simulink library "DQN_Machines"  (R2023b)
settings: Solver=VariableStepAuto  StartTime=0.0  StopTime=10.0  RelTol=1e-3
undefined symbols (not defined in the file): DiscIntNeverNeededParam, N, SM, Ts
libraries: spsabctodq0Lib x2, spsdq0toabcLib x2
(part 3 of 5)

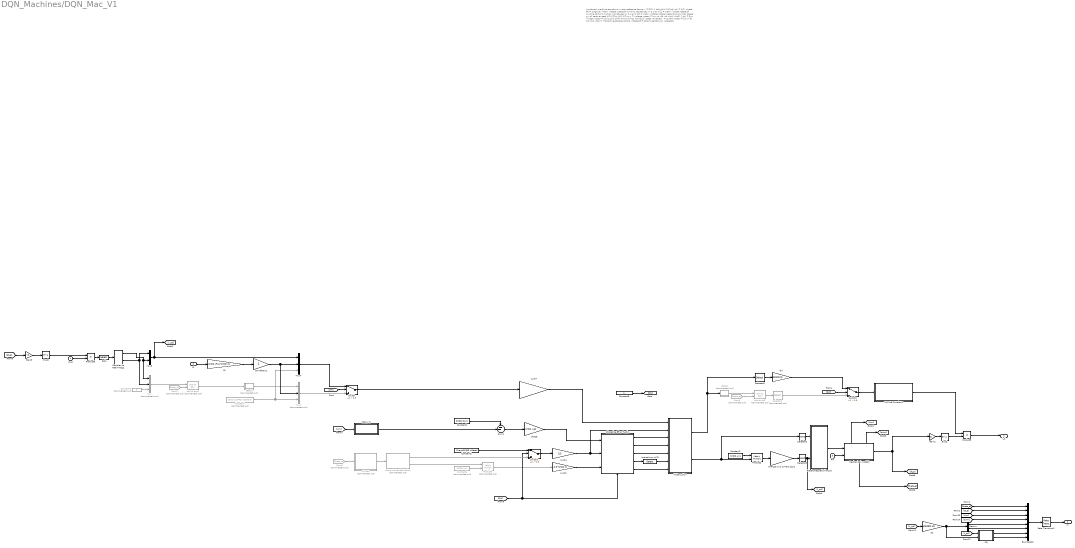
== system DQN_Machines/DQN_Mac_V1 ==
  note: Implement  machine equations in rotor reference frame:
      |   v = [R]*i + dphi/dt + [W]*phi
      | phi = [L]*i
      |
      | where:
      | [R] = diagonal matrix (nState,nState)of winding resistances in d q axis
      | [L] = matrix (nSate,nState)of winding self and mutual inductances in d q axis
      | [W] = matrix (nState,nState) depending on rotor speed wr,
      |       all zeros except W(1,2)=wr  W(2,1)=-wr
      |
      |   v = voltage vector      = [vq   vd   vfd   vkd   vkq1   (vkq2)  ]'
      | phi = flux linkage vector = [phiq phid phifd phikd phikq1 (phikq2)]' (state variables)
      |   i = current vector      = [iq   id   ifd   ikd   ikq1   (ikq2)  ]'
      |
      | if RotorType=Salient-Pole, nState=5
      | if RotorType=Round,        nState=6
  Vs_C : Inport
  Vf : Inport  Port=2
  Pm : Inport  Port=3
  1_Vb1 : Gain  Gain=-0.5*SMRD.Ib  SaturateOnIntegerOverflow=on  OutDataTypeStr=Inherit: Same as input  ParamDataTypeStr=Inherit: Same as input
  1_Vb4 : Gain  Gain=1/3  SaturateOnIntegerOverflow=on  OutDataTypeStr=Inherit: Same as input  ParamDataTypeStr=Inherit: Same as input
  1_Vb7 : Gain  Gain=SMRD.web/SMRD.Vb  SaturateOnIntegerOverflow=on  OutDataTypeStr=Inherit: Same as input  ParamDataTypeStr=Inherit: Same as input
  ABsel2 : Subsystem  Commented=on
  ABsel3 : Subsystem  Commented=on
  Bus Creator : BusCreator  Inputs=8
  Complex to Real-Imag1 : ComplexToRealImag
  Constant : Constant  Commented=on  Value=zeros(1,SMRD.nState-3)
  Constant1 : Constant  Value=SMRD.RLinv
  Constant2 : Constant  Value=3*eye(SMRD.nState)
  Constant4 : Constant  Commented=on  Value=SMRD.Linv
  Constant5 : Constant  Commented=on  Value=0
  Constant7 : Constant  Value=SMRD.Linv
  Constant8 : Constant
  Demux : Demux  Outputs=2
  Discretize BE or Tustin : Subsystem
      settings: PortSchema="{\"entries\":[{\"content\":{\"sides\":[{\"content\":{\"connectorIds\":[\"In1\",\"In2\",\"In3\"]},\"type\":\"ConnectorPlacement.EquallySpacedRectSide\",\"uuid\":\"a6b8bc68-dacc-495a-bf9e-1715fd4ce50f\"},{\"content\":{\"connectorIds\":[\"Out1\",\"Out2\",\"Out3\",\"Out4\",\"Out5\"],\"side\":\"RIGHT\"},\"type\":\"ConnectorPlacement.EquallySpacedRectSide\",\"uuid\":\"950ac892-f5e8-4081-8a8f-99bab3dfce2c\"},{\"content\":{\"side\":\"TOP\"},\"type\":\"ConnectorPlacement.EquallySpacedRectSide\",\"uuid\":\"9af2ed0d-ba89-43cd-9977-15872ca13b39\"},{\"content\":{\"connectorIds\":[\"In4\"],\"side\":\"BOTTOM\"},\"type\":\"ConnectorPlacement.EquallySpacedRectSide\",\"uuid\":\"e70e144b-23c4-40ad-9fe1-8550fd976efc\"}]},\"type\":\"ConnectorPlacement.EquallySpacedConnector\",\"uuid\":\"50b9889c-6d2c-45b1-ad8f-98a7760fa0a3\"}],\"packageUris\":[\"http://schema.mathworks.com/mf0/Connector/R2020b\"],\"version\":\"1.0\"}"
  Electromagnetic Torque : Subsystem
  Exp2 : Math
  Exp3 : Math
  From3 : From  Commented=on  GotoTag=theta_e
  From5 : From  Commented=on  GotoTag=theta_e
  From8 : From  Commented=on  GotoTag=theta_e
  Gain2 : Gain  Gain=1i
  Gain3 : Gain  Gain=-1i
  Ihistory_Flux : Subsystem
  MATLAB Function2 : MATLAB Function  TreatAsAtomicUnit=on  mask{N=SMRD.N}
      mask prompts: N "Harmonic order:"
  Matrix W : Subsystem
      settings: LibrarySourceBlock=spsSynchronousMachineModel/Discrete robust/Matrix W
  Mechanical model1 : Subsystem
      settings: LibrarySourceBlock=spsSynchronousMachineModel/Discrete Pm input trapezoidal  PortSchema="{\"entries\":[{\"content\":{\"sides\":[{\"content\":{\"connectorIds\":[\"In1\",\"In2\"]},\"type\":\"ConnectorPlacement.EquallySpacedRectSide\",\"uuid\":\"2381534f-5abc-4a8d-aa04-ab974f15f8a1\"},{\"content\":{\"connectorIds\":[\"Out1\"],\"side\":\"RIGHT\"},\"type\":\"ConnectorPlacement.EquallySpacedRectSide\",\"uuid\":\"4b91f832-d568-486f-91ee-7f5a07d19f05\"},{\"content\":{\"connectorIds\":[\"Out3\",\"Out4\"],\"side\":\"TOP\"},\"type\":\"ConnectorPlacement.EquallySpacedRectSide\",\"uuid\":\"94f23016-8fd9-49f0-81e0-4b44cc2bc22e\"},{\"content\":{\"connectorIds\":[\"Out2\"],\"side\":\"BOTTOM\"},\"type\":\"ConnectorPlacement.EquallySpacedRectSide\",\"uuid\":\"caf2a10e-4688-4978-a259-17b5afc46c0a\"}]},\"type\":\"ConnectorPlacement.EquallySpacedConnector\",\"uuid\":\"5998548e-4f7b-436e-b4ae-37de4e285cc4\"}],\"packageUris\":[\"http://schema.mathworks.com/mf0/Connector/R2020b\"],\"version\":\"1.0\"}"
  Mux : Mux  Commented=on  Inputs=3
  Mux1 : Mux  Commented=on  Inputs=[2 1 SMRD.nState-3]
  Mux3 : Mux  Inputs=2
  Mux4 : Mux  Inputs=[2 1 SMRD.nState-3]
  N1 : Gain  Gain=SMRD.Vfnp*SMRD.Vb  SaturateOnIntegerOverflow=on  OutDataTypeStr=Inherit: Same as input  ParamDataTypeStr=Inherit: Same as input
  N2 : Gain  Gain=1/SMRD.Vb  SaturateOnIntegerOverflow=on  OutDataTypeStr=Inherit: Same as input  ParamDataTypeStr=Inherit: Same as input
  PQ : Subsystem  AncestorBlock=spsSynchronousMachineModel/Discrete robust/Machine Measurements/PQ
  Product2 : Product  Multiplication=Matrix(*)  SaturateOnIntegerOverflow=on  OutDataTypeStr=Inherit: Same as first input
  Product4 : Product  Commented=on  Multiplication=Matrix(*)  SaturateOnIntegerOverflow=on  OutDataTypeStr=Inherit: Same as first input
  Product5 : Product
  Product6 : Product
  Rate Transition2 : RateTransition  Deterministic=off  OutPortSampleTime=Ts
  SM.VfGain1 : Gain
  Sel1 : Selector  NumberOfDimensions=2  InputPortWidth=3  IndexOptions=Index vector (dialog),Index vector (dialog)  Indices=1,2  OutputSizes=1
  Selector1 : Selector  Commented=on  InputPortWidth=3  IndexOptions=Index vector (dialog)  Indices=[1 2]  OutputSizes=1
  Selector2 : Selector  InputPortWidth=SMRD.nState  IndexOptions=Index vector (dialog)  Indices=[1 2]  OutputSizes=1
  Selector3 : Selector  InputPortWidth=SMRD.nState  IndexOptions=Index vector (dialog)  Indices=[1 2]  OutputSizes=1
  Selector5 : Selector  InputPortWidth=2  IndexOptions=Index vector (dialog)  Indices=[2 1]  OutputSizes=1
  Sum1 : Sum  Inputs=--|  SaturateOnIntegerOverflow=on
  Switch : Switch  Criteria=u2 > Threshold  Threshold=0.5  SaturateOnIntegerOverflow=off  InputSameDT=off
  Switch1 : Switch  Criteria=u2 > Threshold  Threshold=0.5  SaturateOnIntegerOverflow=off  InputSameDT=off
  Switch3 : Switch  Criteria=u2 > Threshold  Threshold=0.5  SaturateOnIntegerOverflow=off  InputSameDT=off
  abc to dq transformation : Subsystem  Commented=on
      settings: LibrarySourceBlock=|
      | spsSynchronousMachineModel/Discrete robust/abc to dq
      | transformation
  abc to dq0 : spsabctodq0Lib/abc to dq0  Commented=on  Alignment=90 degrees behind phase A axis
  change Iq Id current signs : Gain  Gain=SMRD.IqdSign
  dq0 to abc1 : spsdq0toabcLib/dq0 to abc  Commented=on  Alignment=90 degrees behind phase A axis
  ib4 : Gain  Gain=SMRD.Ib  SaturateOnIntegerOverflow=on  OutDataTypeStr=Inherit: Same as input  ParamDataTypeStr=Inherit: Same as input
  last column of D : Selector  NumberOfDimensions=2  InputPortWidth=3  IndexOptions=Index vector (dialog),Index vector (dialog)  Indices=[1:SMRD.nState],3  OutputSizes=1,1
  sin,cos : Subsystem  Commented=on
      settings: LibrarySourceBlock=spsSynchronousMachineModel/Discrete robust/sin,cos
  wbase : Gain  Gain=SMRD.web
  I_C : Outport  VectorParamsAs1DForOutWhenUnconnected=off
  m : Outport  Port=2  VectorParamsAs1DForOutWhenUnconnected=off
  wires:
  Vs_C/1 -> Product6/2  "vd,vq"
  sin,cos/1(sin,cos) -> abc to dq transformation/1(sin,cos)
  1_Vb1/1 -> Discretize BE or Tustin/3(C)
  last column of D/1 -> Ihistory_Flux/6(D(:,3))
  Discretize BE or Tustin/1(Ad) -> Ihistory_Flux/3(Ad)
  Discretize BE or Tustin/4(Dd) -> last column of D/1
  Electromagnetic Torque/1(Te) -> Mechanical model1/1(Te)
  Product2/1 -> change Iq Id current signs/1
  wbase/1 -> Discretize BE or Tustin/1(A)
  Discretize BE or Tustin/5(inv(I_Ts/2*A)) -> Ihistory_Flux/7(inv())
  Discretize BE or Tustin/2(Bd) -> Ihistory_Flux/4(Bd)
  Constant4/1 -> Product4/2  "Linv"
  Matrix W/1("[W]") -> Sum1/2
  Sum1/1 -> wbase/1  "A"
  Product4/1 -> 1_Vb1/1
  Ihistory_Flux/2(phi) -> Product2/2, Selector2/1
  Mechanical model1/2(theta_e) -> [theta_e]
  Mechanical model1/3(we) -> [wm]
  Pm/1 -> Mechanical model1/2(input)
  Constant7/1 -> Product2/1  "Linv"
  Constant2/1 -> Switch1/1
  ABsel3/1(Out1) -> Mux1/1
  Mux1/1 -> Switch/3  "u"
  Constant1/1 -> Sum1/1
  Vf/1 -> N1/1  "Vfd"
  Constant/1 -> Mux1/3, Mux4/3
  SM.VfGain1/1 -> Mux4/2, Mux1/2
  Mux4/1 -> Switch/1  "u"
  N1/1 -> SM.VfGain1/1  "Vfd"
  dq0 to abc1/1 -> ABsel3/1(v)
  abc to dq transformation/2(Ti (2x2)) -> Product4/1
  Switch1/1 -> 1_Vb4/1  "u"
  Ihistory_Flux/1(Ihyst) -> Selector5/1, ABsel2/1(v)  "I(k) = Linv*phi"
  MATLAB Function2/1(Vs_c) -> Product5/1
  Exp2/1 -> Product5/2
  Gain2/1 -> Exp2/1
  Switch/1 -> 1_Vb7/1
  Gain3/1 -> Exp3/1
  [dt_e] -> Gain3/1
  Product6/1 -> Sel1/1
  Exp3/1 -> Product6/1
  Sel1/1 -> Complex to Real-Imag1/1
  Mechanical model1/1(dtheta_e) -> [dt_e], Gain2/1
  Complex to Real-Imag1/2 -> Mux3/1, Mux/2
  Complex to Real-Imag1/1 -> Mux/1, Mux3/2
  Mux3/1 -> [v_qd], Mux4/1
  Switch3/1 -> MATLAB Function2/1(Vdq_vec)
  Mux/1 -> dq0 to abc1/1
  From3/1 -> dq0 to abc1/2
  Constant5/1 -> Mux/3
  1_Vb7/1 -> Ihistory_Flux/1(u)  "u"
  [SW] -> Switch/2
  Constant8/1 -> [SW]
  [SW] -> Switch1/2, Discretize BE or Tustin/4(SW)
  abc to dq transformation/1(Tv (nx3)) -> Switch1/3
  Selector1/1 -> Switch3/3  "Linv"
  [SW] -> Switch3/2
  Selector5/1 -> ib4/1
  abc to dq0/1 -> Selector1/1
  ABsel2/1(I) -> abc to dq0/1
  ib4/1 -> Switch3/1
  From5/1 -> abc to dq0/2
  Product5/1 -> I_C/1
  1_Vb4/1 -> Ihistory_Flux/2(B), Discretize BE or Tustin/2(B)
  [wm] -> Matrix W/1(wr)
  From8/1 -> sin,cos/1(theta)
  Discretize BE or Tustin/3(Cd) -> Ihistory_Flux/5(Cd)
  Bus Creator/1 -> Rate Transition2/1
  [theta_e] -> Bus Creator/1  "Rotor electrical angle  theta (rad)"
  [dt_e] -> Bus Creator/2  "Rotor angle deviation  d_theta (rad)"
  [wm] -> Bus Creator/3  "Rotor speed  wm  (pu)"
  Rate Transition2/1 -> m/1
  [v_qd] -> N2/1
  [i_qd] -> PQ/1(Iqd)
  PQ/1(Peo) -> Bus Creator/7  "Output active power   Peo (pu)"
  PQ/2(Qeo) -> Bus Creator/8  "Output reactive power  Qeo (pu)"
  Mechanical model1/4(dwe) -> [dwm]
  [dwm] -> Bus Creator/4  "Rotor speed deviation  dw (pu)"
  change Iq Id current signs/1 -> Selector3/1
  Selector3/1 -> [i_qd], Electromagnetic Torque/2(iqd)
  Selector2/1 -> Electromagnetic Torque/1(phiqd)
  N2/1 -> PQ/2(Vqd), Demux/1  "Vfd"
  Demux/1 -> Bus Creator/5  "Stator voltage  vq (pu)"
  Demux/2 -> Bus Creator/6  "Stator voltage  vd (pu)"

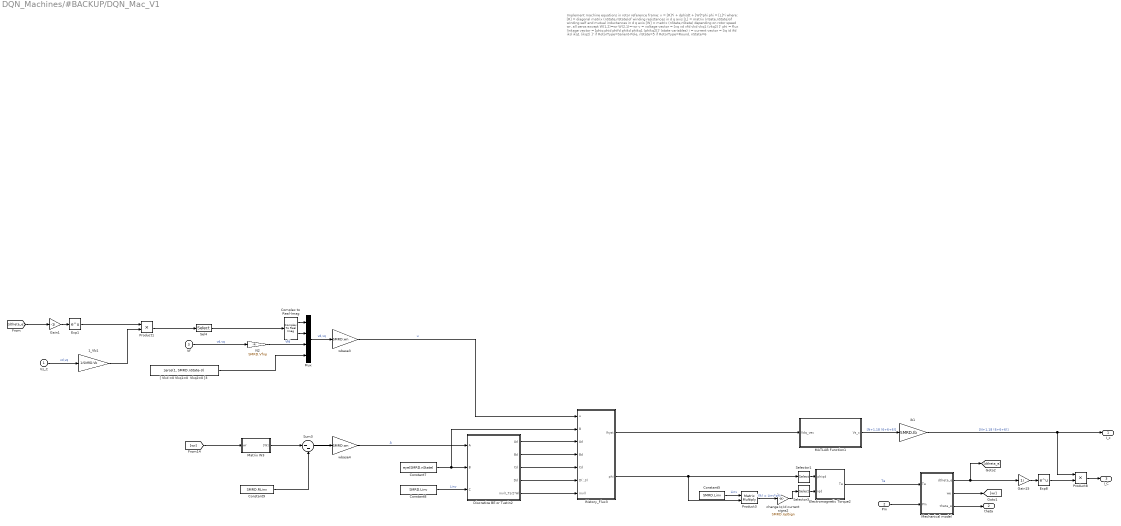
== system DQN_Machines/#BACKUP/DQN_Mac_V1 ==
  note: Implement  machine equations in rotor reference frame:
      |   v = [R]*i + dphi/dt + [W]*phi
      | phi = [L]*i
      |
      | where:
      | [R] = diagonal matrix (nState,nState)of winding resistances in d q axis
      | [L] = matrix (nSate,nState)of winding self and mutual inductances in d q axis
      | [W] = matrix (nState,nState) depending on rotor speed wr,
      |       all zeros except W(1,2)=wr  W(2,1)=-wr
      |
      |   v = voltage vector      = [vq   vd   vfd   vkd   vkq1   (vkq2)  ]'
      | phi = flux linkage vector = [phiq phid phifd phikd phikq1 (phikq2)]' (state variables)
      |   i = current vector      = [iq   id   ifd   ikd   ikq1   (ikq2)  ]'
      |
      | if RotorType=Salient-Pole, nState=5
      | if RotorType=Round,        nState=6
  Vs_C : Inport
  Pm : Inport  Port=2
  Vf : Inport  Port=3
  1_Vb1 : Gain  Gain=1/SMRD.Vb  SaturateOnIntegerOverflow=on  OutDataTypeStr=Inherit: Same as input  ParamDataTypeStr=Inherit: Same as input
  Complex to Real-Imag : ComplexToRealImag
  Constant5 : Constant  Value=SMRD.Linv
  Constant7 : Constant  Value=eye(SMRD.nState)
  Constant8 : Constant  Value=SMRD.Linv
  Constant9 : Constant  Value=SMRD.RLinv
  Discretize BE or Tustin2 : Subsystem  AncestorBlock="spsSynchronousMachineModel/Discrete robust/State Space Model/Discretize  BE or Tustin"
  Electromagnetic Torque2 : Subsystem
  Exp1 : Math
  Exp8 : Math
  Gain1 : Gain  Gain=-1i
  Gain15 : Gain  Gain=1i
  Ihistory_Flux3 : Subsystem  AncestorBlock=spsSynchronousMachineModel/Discrete robust/State Space Model/Ihistory_Flux
  MATLAB Function1 : MATLAB Function  TreatAsAtomicUnit=on  mask{N=SMRD.N}
      mask prompts: N "Harmonic order:"
  Matrix W3 : Subsystem
  Mechanical model : Subsystem
      settings: LibrarySourceBlock=spsSynchronousMachineModel/Discrete Pm input trapezoidal
  Mux : Mux
  N2 : Gain  Gain=SMRD.Vfnp  SaturateOnIntegerOverflow=on  OutDataTypeStr=Inherit: Same as input  ParamDataTypeStr=Inherit: Same as input
  Product1 : Product
  Product3 : Product  Multiplication=Matrix(*)  SaturateOnIntegerOverflow=on  OutDataTypeStr=Inherit: Same as first input
  Product8 : Product
  Sel4 : Selector  NumberOfDimensions=2  InputPortWidth=3  IndexOptions=Index vector (dialog),Index vector (dialog)  Indices=1,2  OutputSizes=1
  Selector1 : Selector  InputPortWidth=SMRD.nState  IndexOptions=Index vector (dialog)  Indices=[1 2]  OutputSizes=1
  Selector3 : Selector  InputPortWidth=SMRD.nState  IndexOptions=Index vector (dialog)  Indices=[1 2]  OutputSizes=1
  Sum3 : Sum  Inputs=|--  SaturateOnIntegerOverflow=on
  "[ Vkd =0 Vkq1=0  Vkq2=0 ]3" : Constant  Value=zeros(1, SMRD.nState-3)
  change Iq Id current signs2 : Gain  Gain=SMRD.IqdSign
  ib1 : Gain  Gain=SMRD.Ib  SaturateOnIntegerOverflow=on  OutDataTypeStr=Inherit: Same as input  ParamDataTypeStr=Inherit: Same as input
  wbase3 : Gain  Gain=SMRD.wn  SaturateOnIntegerOverflow=on  OutDataTypeStr=Inherit: Same as input  ParamDataTypeStr=Inherit: Same as input
  wbase4 : Gain  Gain=SMRD.wn  SaturateOnIntegerOverflow=on  OutDataTypeStr=Inherit: Same as input  ParamDataTypeStr=Inherit: Same as input
  I_c : Outport  VectorParamsAs1DForOutWhenUnconnected=off
  theta : Outport  Port=2  VectorParamsAs1DForOutWhenUnconnected=off
  I_C : Outport  Port=3  VectorParamsAs1DForOutWhenUnconnected=off
  wires:
  Selector3/1 -> Electromagnetic Torque2/2(iqd)
  Constant5/1 -> Product3/1  "Linv"
  Selector1/1 -> Electromagnetic Torque2/1(phiqd)
  Product3/1 -> change Iq Id current signs2/1  "I(k) = Linv*phi"
  Pm/1 -> Mechanical model/2(Pm)
  Electromagnetic Torque2/1(Te) -> Mechanical model/1(Te)  "Te"
  change Iq Id current signs2/1 -> Selector3/1
  MATLAB Function1/1(Vs_c) -> ib1/1  "[N+1,18 (6+6+6)]"
  ib1/1 -> Product8/1, I_c/1  "[N+1,18 (6+6+6)]"
  Sel4/1 -> Complex to Real-Imag/1
  Complex to Real-Imag/2 -> Mux/2
  Complex to Real-Imag/1 -> Mux/1
  N2/1 -> Mux/3  "Vfd"
  Mux/1 -> wbase3/1  "vd,vq"
  Mechanical model/3(theta_e) -> theta/1
  Mechanical model/2(we) -> [wr]
  Vs_C/1 -> 1_Vb1/1  "vd,vq"
  Vf/1 -> N2/1  "vd,vq"
  1_Vb1/1 -> Product1/2
  "[ Vkd =0 Vkq1=0  Vkq2=0 ]3"/1 -> Mux/4
  wbase3/1 -> Ihistory_Flux3/1(u)  "u"
  Discretize BE or Tustin2/4(Dd) -> Ihistory_Flux3/6(D(:,3))
  Discretize BE or Tustin2/5(inv(I_Ts/2*A)) -> Ihistory_Flux3/7(inv())
  Discretize BE or Tustin2/1(Ad) -> Ihistory_Flux3/3(Ad)
  Discretize BE or Tustin2/2(Bd) -> Ihistory_Flux3/4(Bd)
  Discretize BE or Tustin2/3(Cd) -> Ihistory_Flux3/5(Cd)
  Constant7/1 -> Ihistory_Flux3/2(B), Discretize BE or Tustin2/2(B)
  Sum3/1 -> wbase4/1
  Ihistory_Flux3/1(Ihyst) -> MATLAB Function1/1(Vdq_vec)
  Constant8/1 -> Discretize BE or Tustin2/3(C)  "Linv"
  [wr] -> Matrix W3/1(wr)
  Matrix W3/1("[W]") -> Sum3/1
  Constant9/1 -> Sum3/2
  wbase4/1 -> Discretize BE or Tustin2/1(A)  "A"
  Ihistory_Flux3/2(phi) -> Selector1/1, Product3/2
  Gain15/1 -> Exp8/1
  Product8/1 -> I_C/1
  Exp8/1 -> Product8/2
  Gain1/1 -> Exp1/1
  Exp1/1 -> Product1/1
  Product1/1 -> Sel4/1
  Mechanical model/1(dtheta_e) -> [dtheta_e], Gain15/1
  [dtheta_e] -> Gain1/1

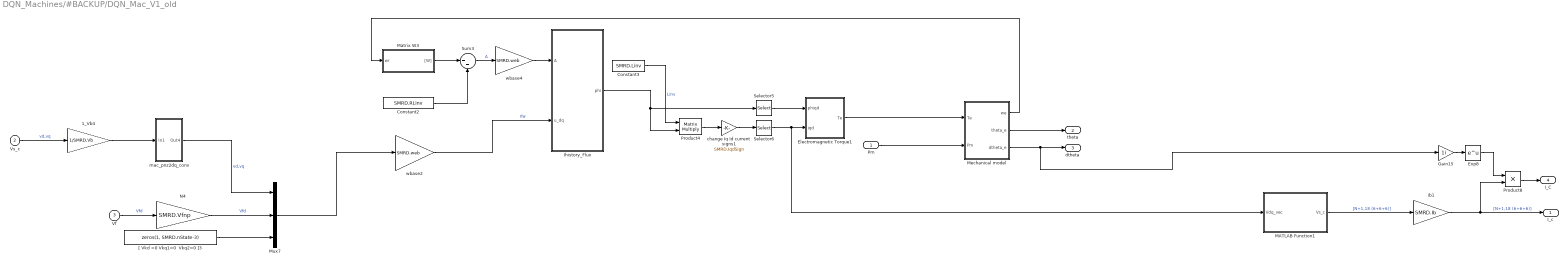
== system DQN_Machines/#BACKUP/DQN_Mac_V1_old ==
  Pm : Inport
  Vs_c : Inport  Port=2
  Vf : Inport  Port=3
  1_Vb4 : Gain  Gain=1/SMRD.Vb  SaturateOnIntegerOverflow=on  OutDataTypeStr=Inherit: Same as input  ParamDataTypeStr=Inherit: Same as input
  Constant2 : Constant  Value=SMRD.RLinv
  Constant3 : Constant  Value=SMRD.Linv
  Electromagnetic Torque1 : Subsystem
  Exp8 : Math
  Gain15 : Gain  Gain=1i
  Ihistory_Flux : Subsystem
  MATLAB Function1 : MATLAB Function  TreatAsAtomicUnit=on  mask{N=HRM}
      mask prompts: N "Harmonic order:"
  Matrix W3 : Subsystem  AncestorBlock=spsSynchronousMachineModel/Discrete robust/Matrix W
  Mechanical model : Subsystem  AncestorBlock=spsSynchronousMachineModel/Discrete Pm input trapezoidal
  Mux7 : Mux  Inputs="[ 2, 1,  (SMRD.nState-3) ]"
  N4 : Gain  Gain=SMRD.Vfnp  SaturateOnIntegerOverflow=on  OutDataTypeStr=Inherit: Same as input  ParamDataTypeStr=Inherit: Same as input
  Product4 : Product  Multiplication=Matrix(*)  SaturateOnIntegerOverflow=on  OutDataTypeStr=Inherit: Same as first input
  Product8 : Product
  Selector5 : Selector  InputPortWidth=SMRD.nState  IndexOptions=Index vector (dialog)  Indices=[1 2]  OutputSizes=1
  Selector6 : Selector  InputPortWidth=SMRD.nState  IndexOptions=Index vector (dialog)  Indices=[1 2]  OutputSizes=1
  Sum3 : Sum  Inputs=|--  SaturateOnIntegerOverflow=on
  "[ Vkd =0 Vkq1=0  Vkq2=0 ]3" : Constant  Value=zeros(1, SMRD.nState-3)
  change Iq Id current signs1 : Gain  Gain=SMRD.IqdSign
  ib1 : Gain  Gain=SMRD.Ib  SaturateOnIntegerOverflow=on  OutDataTypeStr=Inherit: Same as input  ParamDataTypeStr=Inherit: Same as input
  mac_pnz2dq_conv : Subsystem  mask{nrOut=1}
      mask prompts: nrOut "Number of outputs [{C}]"
      mask Display: disp(['{\color{red}\bf\fontsize{12}} [\{X_C\}]',newline,' MUX'], 'texmode','on');
  wbase2 : Gain  Gain=SMRD.web  SaturateOnIntegerOverflow=on  OutDataTypeStr=Inherit: Same as input  ParamDataTypeStr=Inherit: Same as input
  wbase4 : Gain  Gain=SMRD.web
  I_c : Outport  VectorParamsAs1DForOutWhenUnconnected=off
  theta : Outport  Port=2  VectorParamsAs1DForOutWhenUnconnected=off
  dtheta : Outport  Port=3  VectorParamsAs1DForOutWhenUnconnected=off
  I_C : Outport  Port=4  VectorParamsAs1DForOutWhenUnconnected=off
  wires:
  Sum3/1 -> wbase4/1  "A"
  Constant3/1 -> Product4/1  "Linv"
  Matrix W3/1("[W]") -> Sum3/1
  Mechanical model/2(theta_e) -> theta/1
  wbase4/1 -> Ihistory_Flux/1(A)
  Mechanical model/1(we) -> Matrix W3/1(wr)
  Ihistory_Flux/1(phi) -> Product4/2, Selector5/1
  MATLAB Function1/1(Vs_c) -> ib1/1  "[N+1,18 (6+6+6)]"
  Pm/1 -> Mechanical model/2(Pm)
  change Iq Id current signs1/1 -> Selector6/1
  Selector5/1 -> Electromagnetic Torque1/1(phiqd)
  Product4/1 -> change Iq Id current signs1/1
  Constant2/1 -> Sum3/2
  wbase2/1 -> Ihistory_Flux/2(u_dq)  "rlw"
  Electromagnetic Torque1/1(Te) -> Mechanical model/1(Te)
  "[ Vkd =0 Vkq1=0  Vkq2=0 ]3"/1 -> Mux7/3
  Vf/1 -> N4/1  "Vfd"
  Vs_c/1 -> 1_Vb4/1  "vd,vq"
  N4/1 -> Mux7/2  "Vfd"
  1_Vb4/1 -> mac_pnz2dq_conv/1(In1)
  Mux7/1 -> wbase2/1
  mac_pnz2dq_conv/1(Out4) -> Mux7/1  "vd,vq"
  Mechanical model/3(dtheta_e) -> Gain15/1, dtheta/1
  Selector6/1 -> MATLAB Function1/1(Vdq_vec), Electromagnetic Torque1/2(iqd)
  Product8/1 -> I_C/1
  Exp8/1 -> Product8/1
  ib1/1 -> Product8/2, I_c/1  "[N+1,18 (6+6+6)]"
  Gain15/1 -> Exp8/1

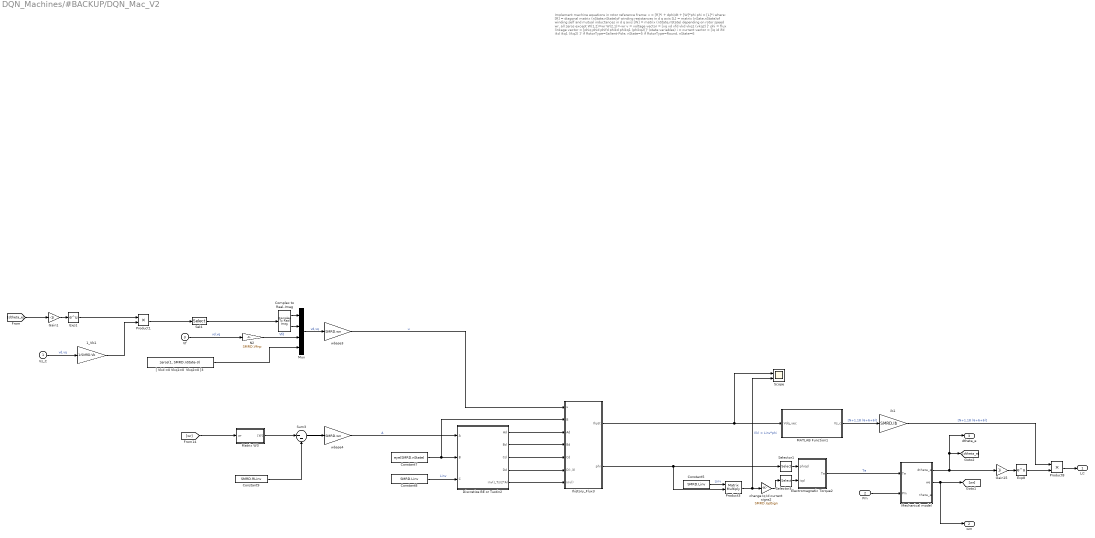
== system DQN_Machines/#BACKUP/DQN_Mac_V2 ==
  note: Implement  machine equations in rotor reference frame:
      |   v = [R]*i + dphi/dt + [W]*phi
      | phi = [L]*i
      |
      | where:
      | [R] = diagonal matrix (nState,nState)of winding resistances in d q axis
      | [L] = matrix (nSate,nState)of winding self and mutual inductances in d q axis
      | [W] = matrix (nState,nState) depending on rotor speed wr,
      |       all zeros except W(1,2)=wr  W(2,1)=-wr
      |
      |   v = voltage vector      = [vq   vd   vfd   vkd   vkq1   (vkq2)  ]'
      | phi = flux linkage vector = [phiq phid phifd phikd phikq1 (phikq2)]' (state variables)
      |   i = current vector      = [iq   id   ifd   ikd   ikq1   (ikq2)  ]'
      |
      | if RotorType=Salient-Pole, nState=5
      | if RotorType=Round,        nState=6
  Vs_C : Inport
  Pm : Inport  Port=2
  Vf : Inport  Port=3
  1_Vb1 : Gain  Gain=1/SMRD.Vb  SaturateOnIntegerOverflow=on  OutDataTypeStr=Inherit: Same as input  ParamDataTypeStr=Inherit: Same as input
  Complex to Real-Imag : ComplexToRealImag
  Constant5 : Constant  Value=SMRD.Linv
  Constant7 : Constant  Value=eye(SMRD.nState)
  Constant8 : Constant  Value=SMRD.Linv
  Constant9 : Constant  Value=SMRD.RLinv
  Discretize BE or Tustin2 : Subsystem  AncestorBlock="spsSynchronousMachineModel/Discrete robust/State Space Model/Discretize  BE or Tustin"
  Electromagnetic Torque2 : Subsystem
  Exp1 : Math
  Exp8 : Math
  Gain1 : Gain  Gain=-1i
  Gain15 : Gain  Gain=1i
  Ihistory_Flux3 : Subsystem  AncestorBlock=spsSynchronousMachineModel/Discrete robust/State Space Model/Ihistory_Flux
  MATLAB Function1 : MATLAB Function  TreatAsAtomicUnit=on  mask{N=SMRD.N}
      mask prompts: N "Harmonic order:"
  Matrix W3 : Subsystem
  Mechanical model : Subsystem
      settings: LibrarySourceBlock=spsSynchronousMachineModel/Discrete Pm input trapezoidal
  Mux : Mux
  N2 : Gain  Gain=SMRD.Vfnp  SaturateOnIntegerOverflow=on  OutDataTypeStr=Inherit: Same as input  ParamDataTypeStr=Inherit: Same as input
  Product1 : Product
  Product3 : Product  Multiplication=Matrix(*)  SaturateOnIntegerOverflow=on  OutDataTypeStr=Inherit: Same as first input
  Product8 : Product
  Scope : Scope  NumInputPorts=2
  Sel4 : Selector  NumberOfDimensions=2  InputPortWidth=3  IndexOptions=Index vector (dialog),Index vector (dialog)  Indices=1,2  OutputSizes=1
  Selector1 : Selector  InputPortWidth=SMRD.nState  IndexOptions=Index vector (dialog)  Indices=[1 2]  OutputSizes=1
  Selector3 : Selector  InputPortWidth=SMRD.nState  IndexOptions=Index vector (dialog)  Indices=[1 2]  OutputSizes=1
  Sum3 : Sum  Inputs=|--  SaturateOnIntegerOverflow=on
  "[ Vkd =0 Vkq1=0  Vkq2=0 ]3" : Constant  Value=zeros(1, SMRD.nState-3)
  change Iq Id current signs2 : Gain  Gain=SMRD.IqdSign
  ib1 : Gain  Gain=SMRD.Ib  SaturateOnIntegerOverflow=on  OutDataTypeStr=Inherit: Same as input  ParamDataTypeStr=Inherit: Same as input
  wbase3 : Gain  Gain=SMRD.wn  SaturateOnIntegerOverflow=on  OutDataTypeStr=Inherit: Same as input  ParamDataTypeStr=Inherit: Same as input
  wbase4 : Gain  Gain=SMRD.wn  SaturateOnIntegerOverflow=on  OutDataTypeStr=Inherit: Same as input  ParamDataTypeStr=Inherit: Same as input
  I_C : Outport  VectorParamsAs1DForOutWhenUnconnected=off
  wm : Outport  Port=2  VectorParamsAs1DForOutWhenUnconnected=off
  dtheta_e : Outport  Port=3  VectorParamsAs1DForOutWhenUnconnected=off
  wires:
  [dtheta_e] -> Gain1/1
  Mechanical model/1(dtheta_e) -> Gain15/1, dtheta_e/1, [dtheta_e]
  Product1/1 -> Sel4/1
  Exp1/1 -> Product1/1
  Gain1/1 -> Exp1/1
  Exp8/1 -> Product8/2
  Product8/1 -> I_C/1
  Gain15/1 -> Exp8/1
  Ihistory_Flux3/2(phi) -> Product3/2, Selector1/1
  wbase4/1 -> Discretize BE or Tustin2/1(A)  "A"
  Constant9/1 -> Sum3/2
  Matrix W3/1("[W]") -> Sum3/1
  [wr] -> Matrix W3/1(wr)
  Constant8/1 -> Discretize BE or Tustin2/3(C)  "Linv"
  Sum3/1 -> wbase4/1
  Constant7/1 -> Discretize BE or Tustin2/2(B), Ihistory_Flux3/2(B)
  Discretize BE or Tustin2/3(Cd) -> Ihistory_Flux3/5(Cd)
  Discretize BE or Tustin2/2(Bd) -> Ihistory_Flux3/4(Bd)
  Discretize BE or Tustin2/1(Ad) -> Ihistory_Flux3/3(Ad)
  Discretize BE or Tustin2/5(inv(I_Ts/2*A)) -> Ihistory_Flux3/7(inv())
  Discretize BE or Tustin2/4(Dd) -> Ihistory_Flux3/6(D(:,3))
  wbase3/1 -> Ihistory_Flux3/1(u)  "u"
  "[ Vkd =0 Vkq1=0  Vkq2=0 ]3"/1 -> Mux/4
  1_Vb1/1 -> Product1/2
  Vf/1 -> N2/1  "vd,vq"
  Vs_C/1 -> 1_Vb1/1  "vd,vq"
  Mechanical model/2(we) -> wm/1, [wr]
  Mux/1 -> wbase3/1  "vd,vq"
  N2/1 -> Mux/3  "Vfd"
  Complex to Real-Imag/1 -> Mux/1
  Complex to Real-Imag/2 -> Mux/2
  Sel4/1 -> Complex to Real-Imag/1
  ib1/1 -> Product8/1  "[N+1,18 (6+6+6)]"
  MATLAB Function1/1(Vs_c) -> ib1/1  "[N+1,18 (6+6+6)]"
  change Iq Id current signs2/1 -> Selector3/1
  Electromagnetic Torque2/1(Te) -> Mechanical model/1(Te)  "Te"
  Pm/1 -> Mechanical model/2(Pm)
  Product3/1 -> Scope/2, change Iq Id current signs2/1  "I(k) = Linv*phi"
  Selector1/1 -> Electromagnetic Torque2/1(phiqd)
  Constant5/1 -> Product3/1  "Linv"
  Selector3/1 -> Electromagnetic Torque2/2(iqd)
  Ihistory_Flux3/1(Ihyst) -> Scope/1, MATLAB Function1/1(Vdq_vec)

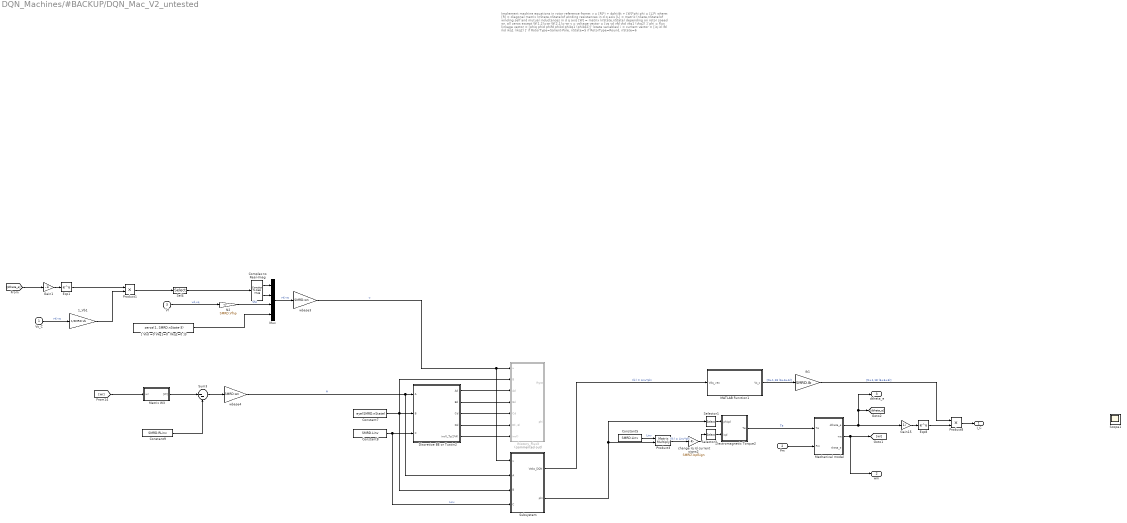
== system DQN_Machines/#BACKUP/DQN_Mac_V2_untested ==
  note: Implement  machine equations in rotor reference frame:
      |   v = [R]*i + dphi/dt + [W]*phi
      | phi = [L]*i
      |
      | where:
      | [R] = diagonal matrix (nState,nState)of winding resistances in d q axis
      | [L] = matrix (nSate,nState)of winding self and mutual inductances in d q axis
      | [W] = matrix (nState,nState) depending on rotor speed wr,
      |       all zeros except W(1,2)=wr  W(2,1)=-wr
      |
      |   v = voltage vector      = [vq   vd   vfd   vkd   vkq1   (vkq2)  ]'
      | phi = flux linkage vector = [phiq phid phifd phikd phikq1 (phikq2)]' (state variables)
      |   i = current vector      = [iq   id   ifd   ikd   ikq1   (ikq2)  ]'
      |
      | if RotorType=Salient-Pole, nState=5
      | if RotorType=Round,        nState=6
  Vs_C : Inport
  Pm : Inport  Port=2
  Vf : Inport  Port=3
  1_Vb1 : Gain  Gain=1/SMRD.Vb  SaturateOnIntegerOverflow=on  OutDataTypeStr=Inherit: Same as input  ParamDataTypeStr=Inherit: Same as input
  Complex to Real-Imag : ComplexToRealImag
  Constant5 : Constant  Value=SMRD.Linv
  Constant7 : Constant  Value=eye(SMRD.nState)
  Constant8 : Constant  Value=SMRD.Linv
  Constant9 : Constant  Value=SMRD.RLinv
  Discretize BE or Tustin2 : Subsystem  AncestorBlock="spsSynchronousMachineModel/Discrete robust/State Space Model/Discretize  BE or Tustin"
  Electromagnetic Torque2 : Subsystem
  Exp1 : Math
  Exp8 : Math
  Gain1 : Gain  Gain=-1i
  Gain15 : Gain  Gain=1i
  Ihistory_Flux3 : Subsystem  Commented=on  AncestorBlock=spsSynchronousMachineModel/Discrete robust/State Space Model/Ihistory_Flux
  MATLAB Function1 : MATLAB Function  TreatAsAtomicUnit=on  mask{N=SMRD.N}
      mask prompts: N "Harmonic order:"
  Matrix W3 : Subsystem
  Mechanical model : Subsystem
      settings: LibrarySourceBlock=spsSynchronousMachineModel/Discrete Pm input trapezoidal
  Mux : Mux
  N2 : Gain  Gain=SMRD.Vfnp  SaturateOnIntegerOverflow=on  OutDataTypeStr=Inherit: Same as input  ParamDataTypeStr=Inherit: Same as input
  Product1 : Product
  Product3 : Product  Multiplication=Matrix(*)  SaturateOnIntegerOverflow=on  OutDataTypeStr=Inherit: Same as first input
  Product8 : Product
  Scope1 : Scope  NumInputPorts=2
  Sel4 : Selector  NumberOfDimensions=2  InputPortWidth=3  IndexOptions=Index vector (dialog),Index vector (dialog)  Indices=1,2  OutputSizes=1
  Selector1 : Selector  InputPortWidth=SMRD.nState  IndexOptions=Index vector (dialog)  Indices=[1 2]  OutputSizes=1
  Selector3 : Selector  InputPortWidth=SMRD.nState  IndexOptions=Index vector (dialog)  Indices=[1 2]  OutputSizes=1
  Subsystem : Subsystem
  Sum3 : Sum  Inputs=|--  SaturateOnIntegerOverflow=on
  "[ Vkd =0 Vkq1=0  Vkq2=0 ]3" : Constant  Value=zeros(1, SMRD.nState-3)
  change Iq Id current signs2 : Gain  Gain=SMRD.IqdSign
  ib1 : Gain  Gain=SMRD.Ib  SaturateOnIntegerOverflow=on  OutDataTypeStr=Inherit: Same as input  ParamDataTypeStr=Inherit: Same as input
  wbase3 : Gain  Gain=SMRD.wn  SaturateOnIntegerOverflow=on  OutDataTypeStr=Inherit: Same as input  ParamDataTypeStr=Inherit: Same as input
  wbase4 : Gain  Gain=SMRD.wn  SaturateOnIntegerOverflow=on  OutDataTypeStr=Inherit: Same as input  ParamDataTypeStr=Inherit: Same as input
  I_C : Outport  VectorParamsAs1DForOutWhenUnconnected=off
  wm : Outport  Port=2  VectorParamsAs1DForOutWhenUnconnected=off
  dtheta_e : Outport  Port=3  VectorParamsAs1DForOutWhenUnconnected=off
  wires:
  Selector3/1 -> Electromagnetic Torque2/2(iqd)
  Constant5/1 -> Product3/1  "Linv"
  Selector1/1 -> Electromagnetic Torque2/1(phiqd)
  Subsystem/1(Vabc_DQN) -> MATLAB Function1/1(Vdq_vec)  "I(k) = Linv*phi"
  Pm/1 -> Mechanical model/2(Pm)
  Electromagnetic Torque2/1(Te) -> Mechanical model/1(Te)  "Te"
  change Iq Id current signs2/1 -> Selector3/1
  MATLAB Function1/1(Vs_c) -> ib1/1  "[N+1,18 (6+6+6)]"
  ib1/1 -> Product8/1  "[N+1,18 (6+6+6)]"
  Sel4/1 -> Complex to Real-Imag/1
  Complex to Real-Imag/2 -> Mux/2
  Complex to Real-Imag/1 -> Mux/1
  N2/1 -> Mux/3  "Vfd"
  Mux/1 -> wbase3/1  "vd,vq"
  Mechanical model/2(we) -> [wr], wm/1
  Vs_C/1 -> 1_Vb1/1  "vd,vq"
  Vf/1 -> N2/1  "vd,vq"
  1_Vb1/1 -> Product1/2
  "[ Vkd =0 Vkq1=0  Vkq2=0 ]3"/1 -> Mux/4
  wbase3/1 -> Subsystem/1(u), Ihistory_Flux3/1(u)  "u"
  Discretize BE or Tustin2/4(Dd) -> Ihistory_Flux3/6(D(:,3))
  Discretize BE or Tustin2/5(inv(I_Ts/2*A)) -> Ihistory_Flux3/7(inv())
  Discretize BE or Tustin2/1(Ad) -> Ihistory_Flux3/3(Ad)
  Discretize BE or Tustin2/2(Bd) -> Ihistory_Flux3/4(Bd)
  Discretize BE or Tustin2/3(Cd) -> Ihistory_Flux3/5(Cd)
  Constant7/1 -> Ihistory_Flux3/2(B), Subsystem/3(B), Discretize BE or Tustin2/2(B)
  Sum3/1 -> wbase4/1
  Constant8/1 -> Subsystem/4(C), Discretize BE or Tustin2/3(C)  "Linv"
  [wr] -> Matrix W3/1(wr)
  Matrix W3/1("[W]") -> Sum3/1
  Constant9/1 -> Sum3/2
  wbase4/1 -> Subsystem/2(A), Discretize BE or Tustin2/1(A)  "A"
  Subsystem/2(phi) -> Selector1/1, Product3/2
  Gain15/1 -> Exp8/1
  Product8/1 -> I_C/1
  Exp8/1 -> Product8/2
  Gain1/1 -> Exp1/1
  Exp1/1 -> Product1/1
  Product1/1 -> Sel4/1
  Mechanical model/1(dtheta_e) -> [dtheta_e], dtheta_e/1, Gain15/1
  [dtheta_e] -> Gain1/1
  Product3/1 -> change Iq Id current signs2/1  "I(k) = Linv*phi"

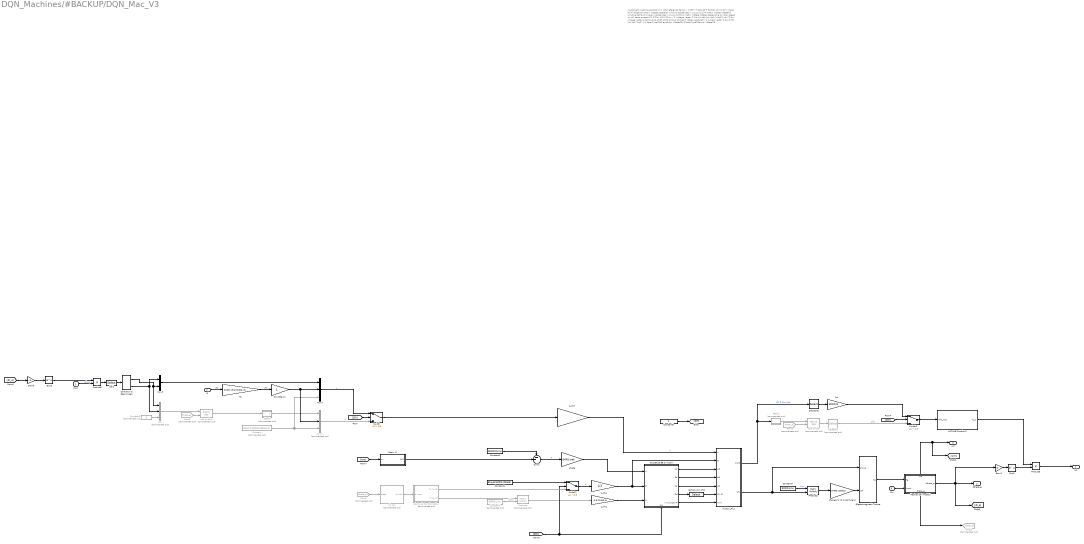
== system DQN_Machines/#BACKUP/DQN_Mac_V3 ==
  note: Implement  machine equations in rotor reference frame:
      |   v = [R]*i + dphi/dt + [W]*phi
      | phi = [L]*i
      |
      | where:
      | [R] = diagonal matrix (nState,nState)of winding resistances in d q axis
      | [L] = matrix (nSate,nState)of winding self and mutual inductances in d q axis
      | [W] = matrix (nState,nState) depending on rotor speed wr,
      |       all zeros except W(1,2)=wr  W(2,1)=-wr
      |
      |   v = voltage vector      = [vq   vd   vfd   vkd   vkq1   (vkq2)  ]'
      | phi = flux linkage vector = [phiq phid phifd phikd phikq1 (phikq2)]' (state variables)
      |   i = current vector      = [iq   id   ifd   ikd   ikq1   (ikq2)  ]'
      |
      | if RotorType=Salient-Pole, nState=5
      | if RotorType=Round,        nState=6
  Vs_C : Inport
  Vf : Inport  Port=2
  Pm : Inport  Port=3
  1_Vb1 : Gain  Gain=-0.5*SMRD.Ib  SaturateOnIntegerOverflow=on  OutDataTypeStr=Inherit: Same as input  ParamDataTypeStr=Inherit: Same as input
  1_Vb4 : Gain  Gain=1/3  SaturateOnIntegerOverflow=on  OutDataTypeStr=Inherit: Same as input  ParamDataTypeStr=Inherit: Same as input
  1_Vb7 : Gain  Gain=SMRD.web/SMRD.Vb  SaturateOnIntegerOverflow=on  OutDataTypeStr=Inherit: Same as input  ParamDataTypeStr=Inherit: Same as input
  ABsel2 : Subsystem  Commented=on
  ABsel3 : Subsystem  Commented=on
  Complex to Real-Imag1 : ComplexToRealImag
  Constant : Constant  Commented=on  Value=zeros(1,SMRD.nState-3)
  Constant1 : Constant  Value=SMRD.RLinv
  Constant2 : Constant  Value=3*eye(SMRD.nState)
  Constant4 : Constant  Commented=on  Value=SMRD.Linv
  Constant5 : Constant  Commented=on  Value=0
  Constant7 : Constant  Value=SMRD.Linv
  Constant8 : Constant
  Discretize BE or Tustin : Subsystem
      settings: PortSchema="{\"entries\":[{\"content\":{\"sides\":[{\"content\":{\"connectorIds\":[\"In1\",\"In2\",\"In3\"]},\"type\":\"ConnectorPlacement.EquallySpacedRectSide\",\"uuid\":\"a6b8bc68-dacc-495a-bf9e-1715fd4ce50f\"},{\"content\":{\"connectorIds\":[\"Out1\",\"Out2\",\"Out3\",\"Out4\",\"Out5\"],\"side\":\"RIGHT\"},\"type\":\"ConnectorPlacement.EquallySpacedRectSide\",\"uuid\":\"950ac892-f5e8-4081-8a8f-99bab3dfce2c\"},{\"content\":{\"side\":\"TOP\"},\"type\":\"ConnectorPlacement.EquallySpacedRectSide\",\"uuid\":\"9af2ed0d-ba89-43cd-9977-15872ca13b39\"},{\"content\":{\"connectorIds\":[\"In4\"],\"side\":\"BOTTOM\"},\"type\":\"ConnectorPlacement.EquallySpacedRectSide\",\"uuid\":\"e70e144b-23c4-40ad-9fe1-8550fd976efc\"}]},\"type\":\"ConnectorPlacement.EquallySpacedConnector\",\"uuid\":\"50b9889c-6d2c-45b1-ad8f-98a7760fa0a3\"}],\"packageUris\":[\"http://schema.mathworks.com/mf0/Connector/R2020b\"],\"version\":\"1.0\"}"
  Electromagnetic Torque : Subsystem
  Exp2 : Math
  Exp3 : Math
  From3 : From  Commented=on  GotoTag=theta_e
  From5 : From  Commented=on  GotoTag=theta_e
  From8 : From  Commented=on  GotoTag=theta_e
  Gain2 : Gain  Gain=1i
  Gain3 : Gain  Gain=-1i
  Goto3 : Goto  Commented=on  GotoTag=theta_e
  Ihistory_Flux : Subsystem
  MATLAB Function2 : MATLAB Function  TreatAsAtomicUnit=on  mask{N=SMRD.N}
      mask prompts: N "Harmonic order:"
  Matrix W : Subsystem
      settings: LibrarySourceBlock=spsSynchronousMachineModel/Discrete robust/Matrix W
  Mechanical model1 : Subsystem
      settings: LibrarySourceBlock=spsSynchronousMachineModel/Discrete Pm input trapezoidal  PortSchema="{\"entries\":[{\"content\":{\"sides\":[{\"content\":{\"connectorIds\":[\"In1\",\"In2\"]},\"type\":\"ConnectorPlacement.EquallySpacedRectSide\",\"uuid\":\"2381534f-5abc-4a8d-aa04-ab974f15f8a1\"},{\"content\":{\"connectorIds\":[\"Out1\"],\"side\":\"RIGHT\"},\"type\":\"ConnectorPlacement.EquallySpacedRectSide\",\"uuid\":\"4b91f832-d568-486f-91ee-7f5a07d19f05\"},{\"content\":{\"connectorIds\":[\"Out3\"],\"side\":\"TOP\"},\"type\":\"ConnectorPlacement.EquallySpacedRectSide\",\"uuid\":\"94f23016-8fd9-49f0-81e0-4b44cc2bc22e\"},{\"content\":{\"connectorIds\":[\"Out2\"],\"side\":\"BOTTOM\"},\"type\":\"ConnectorPlacement.EquallySpacedRectSide\",\"uuid\":\"caf2a10e-4688-4978-a259-17b5afc46c0a\"}]},\"type\":\"ConnectorPlacement.EquallySpacedConnector\",\"uuid\":\"5998548e-4f7b-436e-b4ae-37de4e285cc4\"}],\"packageUris\":[\"http://schema.mathworks.com/mf0/Connector/R2020b\"],\"version\":\"1.0\"}"
  Mux : Mux  Commented=on  Inputs=3
  Mux1 : Mux  Commented=on  Inputs=[2 1 SMRD.nState-3]
  Mux3 : Mux  Inputs=2
  Mux4 : Mux  Inputs=[2 1 SMRD.nState-3]
  N1 : Gain  Gain=SMRD.Vfnp*SMRD.Vb  SaturateOnIntegerOverflow=on  OutDataTypeStr=Inherit: Same as input  ParamDataTypeStr=Inherit: Same as input
  Product2 : Product  Multiplication=Matrix(*)  SaturateOnIntegerOverflow=on  OutDataTypeStr=Inherit: Same as first input
  Product4 : Product  Commented=on  Multiplication=Matrix(*)  SaturateOnIntegerOverflow=on  OutDataTypeStr=Inherit: Same as first input
  Product5 : Product
  Product6 : Product
  SM.VfGain1 : Gain
  Sel1 : Selector  NumberOfDimensions=2  InputPortWidth=3  IndexOptions=Index vector (dialog),Index vector (dialog)  Indices=1,2  OutputSizes=1
  Selector1 : Selector  Commented=on  InputPortWidth=3  IndexOptions=Index vector (dialog)  Indices=[1 2]  OutputSizes=1
  Selector5 : Selector  InputPortWidth=2  IndexOptions=Index vector (dialog)  Indices=[2 1]  OutputSizes=1
  Sum1 : Sum  Inputs=--|  SaturateOnIntegerOverflow=on
  Switch : Switch  Criteria=u2 > Threshold  Threshold=0.5  SaturateOnIntegerOverflow=off  InputSameDT=off
  Switch1 : Switch  Criteria=u2 > Threshold  Threshold=0.5  SaturateOnIntegerOverflow=off  InputSameDT=off
  Switch3 : Switch  Criteria=u2 > Threshold  Threshold=0.5  SaturateOnIntegerOverflow=off  InputSameDT=off
  abc to dq transformation : Subsystem  Commented=on
      settings: LibrarySourceBlock=|
      | spsSynchronousMachineModel/Discrete robust/abc to dq
      | transformation
  abc to dq0 : spsabctodq0Lib/abc to dq0  Commented=on  Alignment=90 degrees behind phase A axis
  change Iq Id current signs : Gain  Gain=SMRD.IqdSign
  dq0 to abc1 : spsdq0toabcLib/dq0 to abc  Commented=on  Alignment=90 degrees behind phase A axis
  ib4 : Gain  Gain=SMRD.Ib  SaturateOnIntegerOverflow=on  OutDataTypeStr=Inherit: Same as input  ParamDataTypeStr=Inherit: Same as input
  last column of D : Selector  NumberOfDimensions=2  InputPortWidth=3  IndexOptions=Index vector (dialog),Index vector (dialog)  Indices=[1:SMRD.nState],3  OutputSizes=1,1
  sin,cos : Subsystem  Commented=on
      settings: LibrarySourceBlock=spsSynchronousMachineModel/Discrete robust/sin,cos
  wbase : Gain  Gain=SMRD.web
  I_C : Outport  VectorParamsAs1DForOutWhenUnconnected=off
  dtheta_e : Outport  Port=2  VectorParamsAs1DForOutWhenUnconnected=off
  wm : Outport  Port=3  VectorParamsAs1DForOutWhenUnconnected=off
  wires:
  Vs_C/1 -> Product6/2  "vd,vq"
  sin,cos/1(sin,cos) -> abc to dq transformation/1(sin,cos)
  1_Vb1/1 -> Discretize BE or Tustin/3(C)
  last column of D/1 -> Ihistory_Flux/6(D(:,3))
  Discretize BE or Tustin/1(Ad) -> Ihistory_Flux/3(Ad)
  Discretize BE or Tustin/4(Dd) -> last column of D/1
  Electromagnetic Torque/1(Te) -> Mechanical model1/1(Te)
  Product2/1 -> change Iq Id current signs/1
  wbase/1 -> Discretize BE or Tustin/1(A)
  Discretize BE or Tustin/5(inv(I_Ts/2*A)) -> Ihistory_Flux/7(inv())
  change Iq Id current signs/1 -> Electromagnetic Torque/2(iqd)
  Discretize BE or Tustin/2(Bd) -> Ihistory_Flux/4(Bd)
  Constant4/1 -> Product4/2  "Linv"
  Matrix W/1("[W]") -> Sum1/2
  Sum1/1 -> wbase/1  "A"
  Product4/1 -> 1_Vb1/1
  Ihistory_Flux/2(phi) -> Product2/2, Electromagnetic Torque/1(phiqd)
  Mechanical model1/2(theta_e) -> Goto3/1
  Mechanical model1/3(we) -> [wm], wm/1
  Pm/1 -> Mechanical model1/2(input)
  Constant7/1 -> Product2/1  "Linv"
  Constant2/1 -> Switch1/1
  ABsel3/1(Out1) -> Mux1/1
  Mux1/1 -> Switch/3  "u"
  Constant1/1 -> Sum1/1
  Vf/1 -> N1/1  "Vfd"
  Constant/1 -> Mux1/3, Mux4/3
  SM.VfGain1/1 -> Mux4/2, Mux1/2
  Mux4/1 -> Switch/1  "u"
  N1/1 -> SM.VfGain1/1  "Vfd"
  dq0 to abc1/1 -> ABsel3/1(v)
  abc to dq transformation/2(Ti (2x2)) -> Product4/1
  Switch1/1 -> 1_Vb4/1  "u"
  Ihistory_Flux/1(Ihyst) -> Selector5/1, ABsel2/1(v)  "I(k) = Linv*phi"
  MATLAB Function2/1(Vs_c) -> Product5/1
  Exp2/1 -> Product5/2
  Gain2/1 -> Exp2/1
  Switch/1 -> 1_Vb7/1
  Gain3/1 -> Exp3/1
  [dt_e] -> Gain3/1
  Product6/1 -> Sel1/1
  Exp3/1 -> Product6/1
  Sel1/1 -> Complex to Real-Imag1/1
  Mechanical model1/1(dtheta_e) -> [dt_e], dtheta_e/1, Gain2/1
  Complex to Real-Imag1/2 -> Mux3/1, Mux/2
  Complex to Real-Imag1/1 -> Mux/1, Mux3/2
  Mux3/1 -> Mux4/1
  Switch3/1 -> MATLAB Function2/1(Vdq_vec)
  Mux/1 -> dq0 to abc1/1
  From3/1 -> dq0 to abc1/2
  Constant5/1 -> Mux/3
  1_Vb7/1 -> Ihistory_Flux/1(u)  "u"
  [SW] -> Switch/2
  Constant8/1 -> [SW]
  [SW] -> Switch1/2, Discretize BE or Tustin/4(SW)
  abc to dq transformation/1(Tv (nx3)) -> Switch1/3
  Selector1/1 -> Switch3/3  "Linv"
  [SW] -> Switch3/2
  Selector5/1 -> ib4/1
  abc to dq0/1 -> Selector1/1
  ABsel2/1(I) -> abc to dq0/1
  ib4/1 -> Switch3/1
  From5/1 -> abc to dq0/2
  Product5/1 -> I_C/1
  1_Vb4/1 -> Ihistory_Flux/2(B), Discretize BE or Tustin/2(B)
  [wm] -> Matrix W/1(wr)
  From8/1 -> sin,cos/1(theta)
  Discretize BE or Tustin/3(Cd) -> Ihistory_Flux/5(Cd)

== system DQN_Machines/DQN_Mac_V1/ABsel2 ==
  v : Inport
  Demux : Demux  Outputs=2
  Mux : Mux  Inputs=3
  Subtract : Sum  Inputs=--
  I : Outport
  wires:
  v/1 -> Demux/1
  Mux/1 -> I/1
  Demux/1 -> Subtract/1, Mux/1
  Demux/2 -> Subtract/2, Mux/2
  Subtract/1 -> Mux/3

== system DQN_Machines/DQN_Mac_V1/ABsel3 ==
  v : Inport
  Demux : Demux  Outputs=3
  Mux : Mux  Inputs=2
  Subtract : Sum  Inputs=+-
  Subtract1 : Sum  Inputs=+-
  Out1 : Outport
  wires:
  v/1 -> Demux/1
  Mux/1 -> Out1/1
  Demux/1 -> Subtract/1
  Demux/2 -> Subtract1/1, Subtract/2
  Subtract/1 -> Mux/1
  Subtract1/1 -> Mux/2
  Demux/3 -> Subtract1/2

== system DQN_Machines/DQN_Mac_V1/Discretize BE or Tustin ==
  note: Implement discretized state-space model using Tustin or TBE method
      |
      | BE      -> SM.DSSmethod=1
      | Tustin  -> SM.DSSmethod=2
      |
      |
      | Tustin
      | ------
      | Ad = inv(I - Ts/2*A)*(I + Ts/2*A)
      | Bd = inv(I - Ts/2*A)*B
      | Cd = C*inv(I - Ts/2*A)*Ts
      | Dd = C*inv(I - Ts/2*A)*B*Ts/2  + D  =  Cd*B/2
      |
      | TBE
      | ---
      | Ad = inv(I - Ts*A)
      | Bd = inv(I - Ts*A)*B
      | Cd = C*inv(I - Ts*A)*Ts
      | Dd = C*inv(I - Ts*A)*B*Ts  + D  =  Cd*B
      |
      | I = eye(SM.nState,SM.nState)
  A : Inport
  B : Inport  Port=2
  C : Inport  Port=3
  SW : Inport  Port=4
  Constant6 : Constant  Value=SMRD.Linv
  Gain : Gain  Gain=-1
  I : Constant  Value=eye(SMRD.nState,SMRD.nState)
  Product1 : Product  Multiplication=Matrix(*)  SaturateOnIntegerOverflow=on  OutDataTypeStr=Inherit: Same as first input
  Product2 : Product  Commented=on  Multiplication=Matrix(*)  SaturateOnIntegerOverflow=on  OutDataTypeStr=Inherit: Same as first input
  Product3 : Product  Multiplication=Matrix(*)  SaturateOnIntegerOverflow=on  OutDataTypeStr=Inherit: Same as first input
  Product4 : Product  Multiplication=Matrix(*)  SaturateOnIntegerOverflow=on  OutDataTypeStr=Inherit: Same as first input
  Sum1 : Sum  Inputs=+-  SaturateOnIntegerOverflow=on
  Sum5 : Sum  SaturateOnIntegerOverflow=on
  Switch2 : Switch  Criteria=u2 > Threshold  Threshold=0.5  SaturateOnIntegerOverflow=off  InputSameDT=off
  "Tustin: 1/2 BE : 1.0" : Gain  Gain=1/2  SaturateOnIntegerOverflow=on  OutDataTypeStr=Inherit: Same as input  ParamDataTypeStr=Inherit: Same as input
  "Tustin: Ts/2 BE : Ts" : Gain  Gain=SMRD.Ts/2  SaturateOnIntegerOverflow=on  OutDataTypeStr=Inherit: Same as input  ParamDataTypeStr=Inherit: Same as input
  inversion : Product  Inputs=/  Multiplication=Matrix(*)  RndMeth=Zero
  wbase3 : Gain  Gain=Ts  SaturateOnIntegerOverflow=on  OutDataTypeStr=Inherit: Same as input  ParamDataTypeStr=Inherit: Same as input
  Ad : Outport  VectorParamsAs1DForOutWhenUnconnected=off
  Bd : Outport  Port=2  VectorParamsAs1DForOutWhenUnconnected=off
  Cd : Outport  Port=3  VectorParamsAs1DForOutWhenUnconnected=off
  Dd : Outport  Port=4  VectorParamsAs1DForOutWhenUnconnected=off
  inv(I_Ts/2*A) : Outport  Port=5  VectorParamsAs1DForOutWhenUnconnected=off
  wires:
  "Tustin: Ts/2 BE : Ts"/1 -> Sum1/2, Sum5/2
  Product4/1 -> Ad/1
  A/1 -> "Tustin: Ts/2 BE : Ts"/1
  I/1 -> Sum5/1, Sum1/1
  Sum1/1 -> inversion/1
  inversion/1 -> Product2/2, Product1/1, Product4/1, inv(I_Ts/2*A)/1
  Sum5/1 -> Product4/2
  Product1/1 -> Bd/1
  B/1 -> Product1/2, Product3/2
  C/1 -> Product2/1
  Product3/1 -> "Tustin: 1/2 BE : 1.0"/1
  "Tustin: 1/2 BE : 1.0"/1 -> Dd/1
  Switch2/1 -> wbase3/1
  Constant6/1 -> Gain/1  "Linv"
  SW/1 -> Switch2/2
  Product2/1 -> Switch2/3
  wbase3/1 -> Cd/1, Product3/1
  Gain/1 -> Switch2/1

== system DQN_Machines/DQN_Mac_V1/Electromagnetic Torque ==
  note: Te computed from stator fluxes and currents
  note: Te=phids*Iqs - phiqs*Ids
  phiqd : Inport
  iqd : Inport  Port=2
  1-1 : Gain  Gain=[1 -1]
  Mult1 : Product  Inputs=**
  Selector1 : Selector  InputPortWidth=2  IndexOptions=Index vector (dialog)  Indices="[2  1]"  OutputSizes=1
  Sum2 : Sum  Inputs=1  SaturateOnIntegerOverflow=on
  Te : Outport  VectorParamsAs1DForOutWhenUnconnected=off
  wires:
  Mult1/1 -> Sum2/1
  1-1/1 -> Mult1/2  "iqs -ids"
  Selector1/1 -> Mult1/1  "phids phiqs"
  Sum2/1 -> Te/1
  phiqd/1 -> Selector1/1
  iqd/1 -> 1-1/1

== system DQN_Machines/DQN_Mac_V1/Ihistory_Flux ==
  u : Inport
  B : Inport  Port=2
  Ad : Inport  Port=3
  Bd : Inport  Port=4
  Cd : Inport  Port=5
  D(:,3) : Inport  Port=6
  inv() : Inport  Port=7
  Add : Sum
  Add1 : Sum
  Add2 : Sum
  BE=1 Tustin=1/2 : Gain  Gain=1/2
  Gain : Gain
  Product{1..2,5..8} (6 alike) : Product  Multiplication=Matrix(*)  SaturateOnIntegerOverflow=on  OutDataTypeStr=Inherit: Same as first input
  Selector4 : Selector  InputPortWidth=SMRD.nState  IndexOptions=Index vector (dialog)  Indices=[1 2]  OutputSizes=1
  Ts : Gain  Gain=Ts  SaturateOnIntegerOverflow=on  OutDataTypeStr=Inherit: Same as input  ParamDataTypeStr=Inherit: Same as input
  Unit Delay : UnitDelay  InitialCondition=SMRD.phidq0/Ts  SampleTime=Ts  HasFrameUpgradeWarning=on
  Vf : Selector  InputPortWidth=SMRD.nState  IndexOptions=Index vector (dialog)  Indices=3  OutputSizes=1
  Ihyst : Outport  VectorParamsAs1DForOutWhenUnconnected=off
  phi : Outport  Port=2  VectorParamsAs1DForOutWhenUnconnected=off
  wires:
  BE=1 Tustin=1/2/1 -> Product8/1
  inv()/1 -> Product6/1
  Cd/1 -> Product2/1
  Ad/1 -> Product5/1
  Add1/1 -> Product6/2
  Product8/1 -> Add1/2
  Product6/1 -> Ts/1
  Product5/1 -> Add/2  "Ad*X"
  Unit Delay/1 -> Product5/2, Add1/1, Product2/2  "xd"
  Add/1 -> Unit Delay/1
  Product1/1 -> Add/1  "Bd*U"
  Product2/1 -> Add2/1
  Add2/1 -> Selector4/1
  Product7/1 -> Add2/2
  Vf/1 -> Product7/2
  D(:,3)/1 -> Product7/1
  u/1 -> Product1/2, Gain/1, Product8/2  "u"
  Bd/1 -> Product1/1  "u"
  B/1 -> BE=1 Tustin=1/2/1  "u"
  Selector4/1 -> Ihyst/1
  Gain/1 -> Vf/1
  Ts/1 -> phi/1

== system DQN_Machines/DQN_Mac_V1/Matrix W ==
  wr : Inport
  Gain1 : Gain  Gain=-1  SaturateOnIntegerOverflow=on  OutDataTypeStr=Inherit: Same as input  ParamDataTypeStr=Inherit: Same as input
  W(1,2)=wr : Assignment  NumberOfDimensions=2  IndexOptions=Index vector (dialog),Index vector (dialog)  Indices=1,2  OutputSizes=1,1
  W(2,1)=-wr : Assignment  NumberOfDimensions=2  IndexOptions=Index vector (dialog),Index vector (dialog)  Indices=2,1  OutputSizes=1,1
  u1 : Constant  Value=zeros(SMRD.nState,SMRD.nState)
  "[W]" : Outport  VectorParamsAs1DForOutWhenUnconnected=off
  wires:
  u1/1 -> W(1,2)=wr/1
  Gain1/1 -> W(2,1)=-wr/2
  W(1,2)=wr/1 -> W(2,1)=-wr/1
  wr/1 -> W(1,2)=wr/2, Gain1/1
  W(2,1)=-wr/1 -> "[W]"/1

== system DQN_Machines/DQN_Mac_V1/Mechanical model1 ==
  note: *
  Te : Inport  PortDimensions=1
  input : Inport  Port=2
  1 ----- 2H : Gain  Gain=1/(2*SMRD.H)  SaturateOnIntegerOverflow=on  OutDataTypeStr=Inherit: Same as input  ParamDataTypeStr=Inherit: Same as input
  1_Pb : Gain  Gain=1/SMRD.Pb  SaturateOnIntegerOverflow=on  OutDataTypeStr=Inherit: Same as input  ParamDataTypeStr=Inherit: Same as input
  Delay Prediction : Subsystem
  Digital Clock : DigitalClock  SampleTime=SMRD.Ts
  F : Gain  Gain=SMRD.F  SaturateOnIntegerOverflow=on  OutDataTypeStr=Inherit: Same as input  ParamDataTypeStr=Inherit: Same as input
  Mux1 : Mux  Inputs=2
  Rate Transition1 : RateTransition  Deterministic=off  OutPortSampleTime=Ts
  Rotor angle dthetae : DiscreteIntegrator  InitialCondition=SMRD.tho  SampleTime=SMRD.Ts  ICPrevOutput=DiscIntNeverNeededParam  ICPrevScaledInput=DiscIntNeverNeededParam
  Rotor speed deviation (dw) : DiscreteIntegrator  IntegratorMethod=Integration: Trapezoidal  InitialCondition=SMRD.dwo  SampleTime=SMRD.Ts  ICPrevOutput=DiscIntNeverNeededParam  ICPrevScaledInput=DiscIntNeverNeededParam
  Sum : Sum  InputSameDT=on  SaturateOnIntegerOverflow=on  OutDataTypeStr=Inherit: Same as first input
  Sum2 : Sum  Inputs=+--  InputSameDT=on  SaturateOnIntegerOverflow=on  OutDataTypeStr=Inherit: Same as first input
  Sum3 : Sum  InputSameDT=on  SaturateOnIntegerOverflow=on  OutDataTypeStr=Inherit: Same as first input
  div : Fcn  Expr=u[2]/u[1]
      mask Display: disp('/')
  nominal speed : Constant
  we base : Gain  Gain=SMRD.web  SaturateOnIntegerOverflow=on  OutDataTypeStr=Inherit: Same as input  ParamDataTypeStr=Inherit: Same as input
  web2 : Gain  Gain=SMRD.web  SaturateOnIntegerOverflow=on  OutDataTypeStr=Inherit: Same as input  ParamDataTypeStr=Inherit: Same as input
  dtheta_e : Outport  InitialOutput=0  VectorParamsAs1DForOutWhenUnconnected=off
  theta_e : Outport  Port=2  InitialOutput=0  VectorParamsAs1DForOutWhenUnconnected=off
  we : Outport  Port=3  InitialOutput=0  VectorParamsAs1DForOutWhenUnconnected=off
  dwe : Outport  Port=4  InitialOutput=0  VectorParamsAs1DForOutWhenUnconnected=off
  wires:
  Delay Prediction/1(dw) -> dwe/1, we base/1, Sum/2  "dw"
  Rate Transition1/1 -> 1_Pb/1
  Rotor angle dthetae/1 -> Sum3/1, dtheta_e/1  "d_theta (rad)"
  web2/1 -> Sum3/2
  Digital Clock/1 -> web2/1
  we base/1 -> Rotor angle dthetae/1
  Rotor speed deviation (dw)/1 -> Delay Prediction/1(in)  "dw"
  nominal speed/1 -> Sum/1
  1 ----- 2H/1 -> Rotor speed deviation (dw)/1
  div/1 -> Sum2/1
  Te/1 -> Sum2/2  "Te"
  Mux1/1 -> div/1
  input/1 -> Rate Transition1/1  "Pm"
  1_Pb/1 -> Mux1/2
  F/1 -> Sum2/3
  Sum2/1 -> 1 ----- 2H/1
  Sum/1 -> F/1, we/1, Mux1/1  "n"
  Sum3/1 -> theta_e/1

== system DQN_Machines/DQN_Mac_V1/PQ ==
  note: PQ Measurement:
  note: Q = Vq*Id-Vd*Iq
  note: P = Vd*Id + Vq*Iq
  Iqd : Inport
  Vqd : Inport  Port=2
  Demux : Demux  Outputs=2
  Demux1 : Demux  Outputs=[1,1]
      settings: DisplayOption=none
  Gain : Gain  SaturateOnIntegerOverflow=on  OutDataTypeStr=Inherit: Same as input  ParamDataTypeStr=Inherit: Same as input
  Gain1 : Gain  SaturateOnIntegerOverflow=on  OutDataTypeStr=Inherit: Same as input  ParamDataTypeStr=Inherit: Same as input
  Product{2..5} (4 alike) : Product  InputSameDT=on  SaturateOnIntegerOverflow=on  OutDataTypeStr=Inherit: Same as first input
  Sum : Sum  InputSameDT=on  SaturateOnIntegerOverflow=on  OutDataTypeStr=Inherit: Same as first input
  Sum1 : Sum  Inputs=+-  InputSameDT=on  SaturateOnIntegerOverflow=on  OutDataTypeStr=Inherit: Same as first input
  Peo : Outport  VectorParamsAs1DForOutWhenUnconnected=off
  Qeo : Outport  Port=2  VectorParamsAs1DForOutWhenUnconnected=off
  wires:
  Demux1/2 -> Product4/2, Product3/2
  Demux/1 -> Product4/1, Product2/1
  Demux/2 -> Product5/1, Product3/1
  Sum1/1 -> Gain1/1  "Qeo"
  Sum/1 -> Gain/1  "Peo"
  Product5/1 -> Sum1/2
  Product4/1 -> Sum1/1
  Product3/1 -> Sum/2
  Product2/1 -> Sum/1
  Gain/1 -> Peo/1
  Gain1/1 -> Qeo/1
  Iqd/1 -> Demux1/1
  Demux1/1 -> Product2/2, Product5/2
  Vqd/1 -> Demux/1
